simulink model "sampleModel1906"  (R2023a)
settings: Solver=VariableStepAuto  StartTime=0.0  StopTime=10.0  RelTol=1e-3
libraries: hdlsllib x4, simulink x2
settings Model: Creator=user1  LastModifiedBy=user1

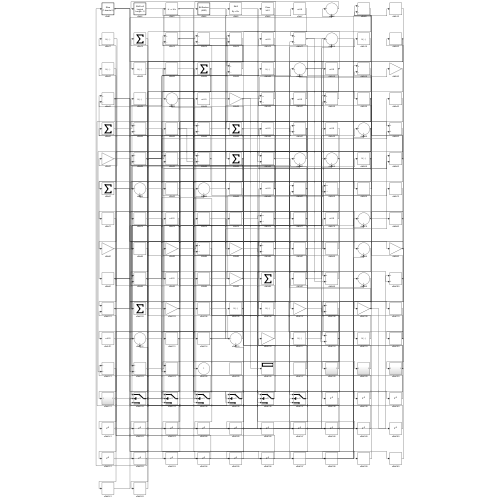
[thumbnail: Simulink's stored preview of the top-level diagram]
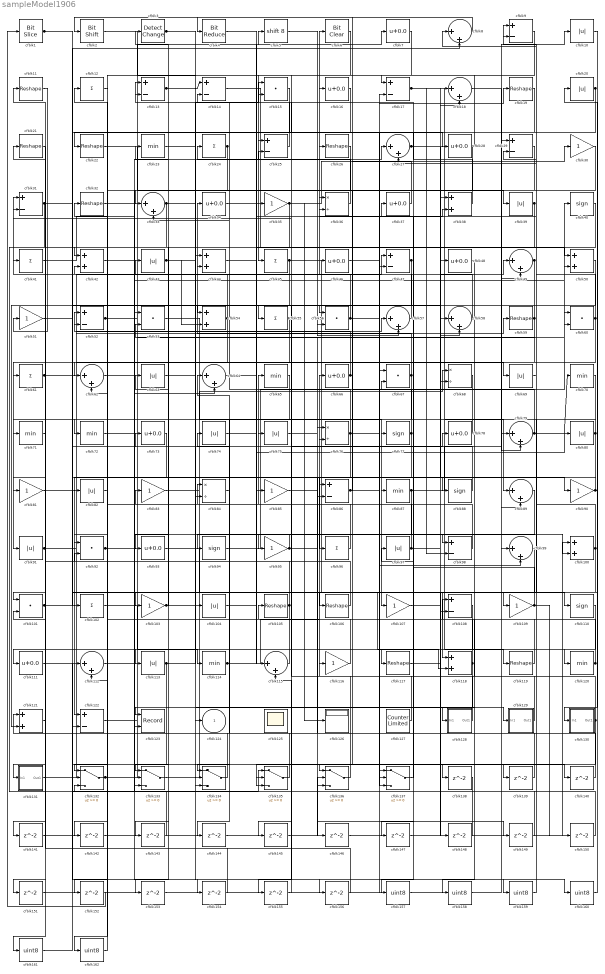
== system sampleModel1906 ==
  cfblk1 : hdlsllib/Logic and Bit Operations/Bit Slice  lidx=7  ridx=0
  cfblk{10,20,39,43,63,69,74..75,80,82,91,97,104,113} (14 alike) : Abs  SaturateOnIntegerOverflow=off
  cfblk{38,42,44,50,54,100,118,121} (8 alike) : Sum
  cfblk{15,53,56,60,67,92,101} (7 alike) : DotProduct  OutDataTypeStr=Inherit: Inherit via internal rule
  cfblk{12,24,41,45,55,61,96,102} (8 alike) : Sum  Inputs=+
  cfblk{30,35,51,81,83,85,90,95,103,107,109,116} (12 alike) : Gain
  cfblk{11,19,21..22,26,32,59,105..106,117,119} (11 alike) : Reshape
  cfblk{9,13..14,17,25,29,31,47,52,86,98,108,122} (13 alike) : Sum  Inputs=+-
  cfblk{40,77,88,94,110} (5 alike) : Signum
  cfblk{7,16,28,34,37,46,48,66,73,78,93,111} (12 alike) : Bias  Bias=0.0  SaturateOnIntegerOverflow=off
  cfblk{8,18,27,33,49,57..58,62,64,79,89,99,112,115} (14 alike) : Sum  Inputs=|++
  cfblk{23,65,70..72,87,114,120} (8 alike) : MinMax
  cfblk123 : Record  FileSettingsInternal="{\"entries\":[{\"content\":{\"excelSettings\":{\"content\":{},\"type\":\"Streamout.ExcelSettings\"}},\"type\":\"Streamout.FileSettingStorage\",\"uuid\":\"\"}],\"packageUris\":[\"http:\\/\\/schema.mathworks.com\\/mf0\\/streamout_blocks\\/R2020a\"],\"version\":\"1.0\"}"  Layout=[1 1]  SignalsInternal="{\"entries\":[{\"content\":{\"signals\":[{\"content\":{\"blockPath\":[],\"dimensions\":[1],\"domain\":\"\",\"lineColor\":\"#a2142f\",\"plots\":[1],\"port\":1,\"signalID\":5065,\"signalName\":\"XY Graph:1\"},\"type\":\"RecordBlkView.Signal\",\"uuid\":\"\"},{\"content\":{\"blockPath\":[],\"dimensions\":[1],\"domain\":\"\",\"lineColor\":\"#139fff\",\"plots\":[1],\"port\":2,\"signalID\":5068,\"signalName\":\"XY Graph:2\"},\"type\":\"RecordBlkView.Signal\",\"uuid\":\"\"}]},\"type\":\"RecordBlkView.InputSignals\",\"uuid\":\"\"}],\"packageUris\":[\"http:\\/\\/schema.mathworks.com\\/mf0\\/streamout_blocks\\/R2020a\"],\"version\":\"1.0\"}"  VisualizationBindings="{\"xyplotplugin\":{\"info\":[{\"series\":[{\"bindingParametersList\":[{\"parameter\":\"X-Axis\",\"signalID\":5065,\"signalName\":\"XY Graph:1\"},{\"parameter\":\"Y-Axis\",\"signalID\":5068,\"signalName\":\"XY Graph:2\"}],\"seriesID\":46358}],\"subplotID\":1}]}}"  CompatibilityTag=XY  st=-1
  cfblk125 : Scope
      settings: Floating=on
  cfblk126 : Display
  cfblk127 : hdlsllib/Sources/Counter Limited  uplimit=7  tsamp=-1
  cfblk128 : Subsystem
      settings: LibrarySourceBlock=|
      | hdlsllib/Ports &
      | Subsystems/Subsystem
  cfblk129 : Subsystem
      settings: LibrarySourceBlock=|
      | hdlsllib/Ports &
      | Subsystems/Subsystem
  cfblk130 : Subsystem
      settings: LibrarySourceBlock=|
      | hdlsllib/Ports &
      | Subsystems/Subsystem
  cfblk131 : Subsystem
      settings: LibrarySourceBlock=|
      | hdlsllib/Ports &
      | Subsystems/Subsystem
  cfblk{132..137} (6 alike) : Switch  SaturateOnIntegerOverflow=off  InputSameDT=off
  cfblk{138..156} (19 alike) : Delay  SampleTime=1
  cfblk{157..162} (6 alike) : DataTypeConversion  OutDataTypeStr=uint8  SaturateOnIntegerOverflow=off  RndMeth=Floor
  cfblk2 : hdlsllib/Logic and Bit Operations/Bit Shift  mode=Shift Left Logical  N=0
  cfblk3 : simulink/Logic and Bit Operations/Detect Change  vinit=0  OutDataTypeStr=boolean
      settings: LibrarySourceBlock=|
      | hdlsllib/Logic and Bit
      | Operations/Detect
      | Change
  cfblk{36,68,76,84} (4 alike) : Product  Inputs=*/  RndMeth=Zero  SaturateOnIntegerOverflow=on
  cfblk4 : hdlsllib/Logic and Bit Operations/Bit Reduce  mode=AND
  cfblk5 : ArithShift  BitShiftNumber=8
  cfblk6 : simulink/Logic and Bit Operations/Bit Clear  iBit=0
      settings: LibrarySourceBlock=|
      | hdlsllib/Logic and Bit
      | Operations/Bit Clear
  cfblk124 : Outport  VectorParamsAs1DForOutWhenUnconnected=off
  wires:
  cfblk122/1 -> cfblk5/1
  cfblk116/1 -> cfblk105/1
  cfblk110/1 -> cfblk120/1
  cfblk56/1 -> cfblk6/1, cfblk99/2
  cfblk134/1 -> cfblk73/1
  cfblk67/1 -> cfblk34/1, cfblk134/1
  cfblk55/1 -> cfblk91/1, cfblk134/3
  cfblk68/1 -> cfblk107/1
  cfblk97/1 -> cfblk65/1, cfblk18/2
  cfblk101/1 -> cfblk59/1, cfblk75/1
  cfblk37/1 -> cfblk2/1
  cfblk10/1 -> cfblk118/1
  cfblk17/1 -> cfblk119/1, cfblk98/2
  cfblk81/1 -> cfblk57/1
  cfblk31/1 -> cfblk135/1, cfblk84/2, cfblk86/2
  cfblk28/1 -> cfblk17/1, cfblk133/2
  cfblk111/1 -> cfblk43/1
  cfblk35/1 -> cfblk30/1, cfblk126/1, cfblk103/1
  cfblk91/1 -> cfblk78/1, cfblk108/2, cfblk8/2
  cfblk36/1 -> cfblk24/1
  cfblk8/1 -> cfblk4/1
  cfblk94/1 -> cfblk40/1
  cfblk49/1 -> cfblk55/1, cfblk121/2
  cfblk78/1 -> cfblk72/1
  cfblk93/1 -> cfblk118/2
  cfblk137/1 -> cfblk97/1
  cfblk128/1(Out1) -> cfblk52/1
  cfblk45/1 -> cfblk110/1, cfblk61/1
  cfblk27/1 -> cfblk89/1, cfblk90/1
  cfblk133/1 -> cfblk68/1
  cfblk120/1 -> cfblk117/1, cfblk42/2
  cfblk131/1(Out1) -> cfblk58/1
  cfblk114/1 -> cfblk66/1, cfblk38/2
  cfblk5/1 -> cfblk57/2
  cfblk64/1 -> cfblk7/1
  cfblk42/1 -> cfblk87/1
  cfblk86/1 -> cfblk16/1, cfblk98/1
  cfblk135/1 -> cfblk121/1
  cfblk25/1 -> cfblk13/1
  cfblk61/1 -> cfblk69/1, cfblk154/1
  cfblk98/1 -> cfblk32/1
  cfblk102/1 -> cfblk114/1
  cfblk79/1 -> cfblk70/1, cfblk36/2
  cfblk7/1 -> cfblk45/1
  cfblk113/1 -> cfblk15/1, cfblk133/3
  cfblk73/1 -> cfblk122/1
  cfblk80/1 -> cfblk71/1, cfblk96/1
  cfblk23/1 -> cfblk44/1
  cfblk3/1 -> cfblk56/1, cfblk129/1(In1)
  cfblk130/1(Out1) -> cfblk44/2, cfblk135/2, cfblk116/1
  cfblk14/1 -> cfblk137/1
  cfblk43/1 -> cfblk104/1, cfblk54/2
  cfblk11/1 -> cfblk51/1
  cfblk53/1 -> cfblk77/1
  cfblk132/1 -> cfblk48/1, cfblk64/2
  cfblk136/1 -> cfblk76/2
  cfblk52/1 -> cfblk46/1, cfblk27/1, cfblk25/2, cfblk47/1
  cfblk115/1 -> cfblk111/1
  cfblk4/1 -> cfblk85/1
  cfblk100/1 -> cfblk128/1(In1), cfblk27/2
  cfblk118/1 -> cfblk84/1, cfblk143/1
  cfblk2/1 -> cfblk124/1
  cfblk19/1 -> cfblk92/1
  cfblk33/1 -> cfblk131/1(In1), cfblk86/1, cfblk137/3
  cfblk92/1 -> cfblk67/1, cfblk50/2
  cfblk72/1 -> cfblk100/2
  cfblk99/1 -> cfblk122/2
  cfblk66/1 -> cfblk136/1, cfblk12/1, cfblk23/1
  cfblk117/1 -> cfblk49/1
  cfblk26/1 -> cfblk33/1
  cfblk40/1 -> cfblk113/1
  cfblk21/1 -> cfblk81/1
  cfblk32/1 -> cfblk68/2
  cfblk30/1 -> cfblk106/1
  cfblk41/1 -> cfblk26/1
  cfblk119/1 -> cfblk74/1
  cfblk71/1 -> cfblk101/1
  cfblk34/1 -> cfblk35/1
  cfblk127/1 -> cfblk31/1
  cfblk13/1 -> cfblk14/1, cfblk88/1
  cfblk24/1 -> cfblk42/1, cfblk142/1
  cfblk54/1 -> cfblk93/1, cfblk41/1
  cfblk9/1 -> cfblk62/1
  cfblk62/1 -> cfblk60/1
  cfblk20/1 -> cfblk47/2, cfblk147/1
  cfblk18/1 -> cfblk79/2
  cfblk50/1 -> cfblk56/2
  cfblk104/1 -> cfblk80/1
  cfblk15/1 -> cfblk22/1
  cfblk95/1 -> cfblk94/1, cfblk149/1
  cfblk77/1 -> cfblk132/1, cfblk67/2
  cfblk105/1 -> cfblk21/1, cfblk161/1
  cfblk6/1 -> cfblk25/1
  cfblk89/1 -> cfblk136/3
  cfblk75/1 -> cfblk60/2
  cfblk58/1 -> cfblk31/2, cfblk158/1
  cfblk39/1 -> cfblk123/1, cfblk123/2
  cfblk76/1 -> cfblk19/1, cfblk33/2, cfblk134/2
  cfblk38/1 -> cfblk13/2
  cfblk44/1 -> cfblk50/1
  cfblk60/1 -> cfblk36/1, cfblk8/1, cfblk162/1
  cfblk83/1 -> cfblk38/1
  cfblk109/1 -> cfblk9/1, cfblk37/1, cfblk150/1
  cfblk70/1 -> cfblk109/1
  cfblk74/1 -> cfblk115/1
  cfblk88/1 -> cfblk15/2
  cfblk90/1 -> cfblk82/1, cfblk130/1(In1)
  cfblk87/1 -> cfblk10/1, cfblk145/1
  cfblk57/1 -> cfblk14/2
  cfblk103/1 -> cfblk83/1, cfblk159/1
  cfblk1/1 -> cfblk28/1, cfblk135/3, cfblk58/2
  cfblk82/1 -> cfblk102/1
  cfblk69/1 -> cfblk9/2
  cfblk106/1 -> cfblk63/1
  cfblk16/1 -> cfblk62/2
  cfblk22/1 -> cfblk39/1
  cfblk47/1 -> cfblk133/1, cfblk95/1
  cfblk96/1 -> cfblk3/1
  cfblk59/1 -> cfblk53/2, cfblk54/1, cfblk155/1
  cfblk129/1(Out1) -> cfblk108/1
  cfblk48/1 -> cfblk138/1
  cfblk138/1 -> cfblk132/3
  cfblk46/1 -> cfblk139/1
  cfblk139/1 -> cfblk64/1
  cfblk63/1 -> cfblk140/1
  cfblk140/1 -> cfblk76/1
  cfblk65/1 -> cfblk141/1
  cfblk141/1 -> cfblk89/2
  cfblk142/1 -> cfblk136/2
  cfblk143/1 -> cfblk53/1
  cfblk84/1 -> cfblk144/1
  cfblk144/1 -> cfblk18/1
  cfblk145/1 -> cfblk137/2
  cfblk85/1 -> cfblk146/1
  cfblk146/1 -> cfblk100/1
  cfblk147/1 -> cfblk79/1
  cfblk107/1 -> cfblk148/1
  cfblk148/1 -> cfblk132/2
  cfblk149/1 -> cfblk52/2
  cfblk150/1 -> cfblk92/2
  cfblk121/1 -> cfblk151/1
  cfblk151/1 -> cfblk49/2
  cfblk12/1 -> cfblk152/1
  cfblk152/1 -> cfblk1/1
  cfblk108/1 -> cfblk153/1
  cfblk153/1 -> cfblk17/2
  cfblk154/1 -> cfblk101/2
  cfblk155/1 -> cfblk115/2
  cfblk51/1 -> cfblk156/1
  cfblk156/1 -> cfblk11/1
  cfblk29/1 -> cfblk157/1
  cfblk157/1 -> cfblk99/1
  cfblk158/1 -> cfblk29/1
  cfblk159/1 -> cfblk29/2
  cfblk112/1 -> cfblk160/1
  cfblk160/1 -> cfblk20/1
  cfblk161/1 -> cfblk112/1
  cfblk162/1 -> cfblk112/2

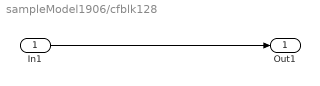
== system sampleModel1906/cfblk128 ==
  In1 : Inport
  Out1 : Outport
  wires:
  In1/1 -> Out1/1

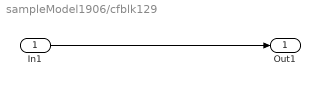
== system sampleModel1906/cfblk129 ==
  In1 : Inport
  Out1 : Outport
  wires:
  In1/1 -> Out1/1

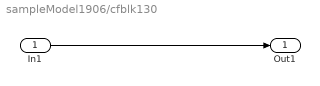
== system sampleModel1906/cfblk130 ==
  In1 : Inport
  Out1 : Outport
  wires:
  In1/1 -> Out1/1

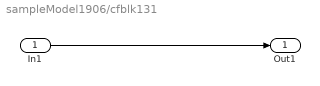
== system sampleModel1906/cfblk131 ==
  In1 : Inport
  Out1 : Outport
  wires:
  In1/1 -> Out1/1
